simulink model "PDischargeDerate"  (R2024b)
settings: configuration reference "STM32H7_Config" (kept outside this file)
settings Model: DataDictionary=Master_Dictionary.sldd  EnableAccessToBaseWorkspace=off  Creator=torni  LastModifiedBy=Will
settings ConfigSetRef: SourceName=STM32H7_Config

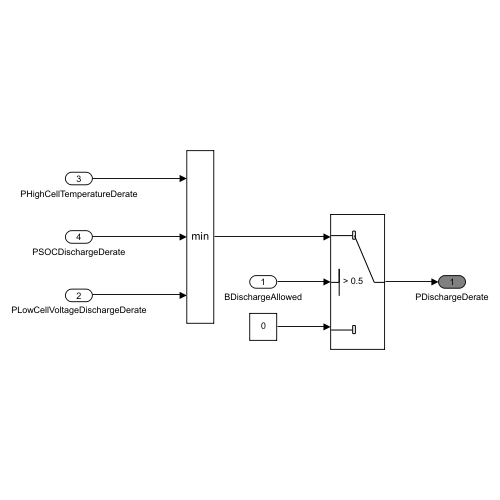
[thumbnail: Simulink's stored preview of the top-level diagram]
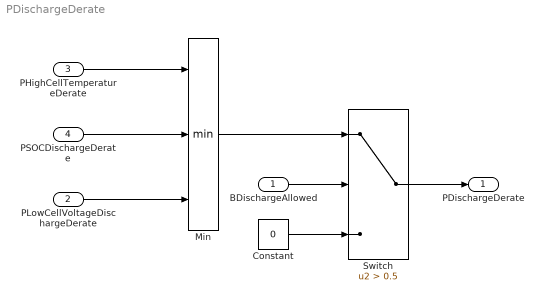
== system PDischargeDerate ==
  "BDischargeAllowed " : Inport  OutDataTypeStr=boolean
  PLowCellVoltageDischargeDerate : Inport  Port=2  OutDataTypeStr=double
  PHighCellTemperatureDerate : Inport  Port=3  OutDataTypeStr=double
  PSOCDischargeDerate : Inport  Port=4  OutDataTypeStr=double
  Constant : Constant  Value=0
  Min : MinMax  Inputs=3
  Switch : Switch  Criteria=u2 > Threshold  Threshold=0.5  SaturateOnIntegerOverflow=off  InputSameDT=off
  PDischargeDerate : Outport  OutDataTypeStr=double  VectorParamsAs1DForOutWhenUnconnected=off
  wires:
  Constant/1 -> Switch/3
  Min/1 -> Switch/1
  Switch/1 -> PDischargeDerate/1
  "BDischargeAllowed "/1 -> Switch/2
  PLowCellVoltageDischargeDerate/1 -> Min/3
  PSOCDischargeDerate/1 -> Min/2
  PHighCellTemperatureDerate/1 -> Min/1
